simulink model "boost_converter"  (R2013a)
settings: Solver=ode23tb  StartTime=0.0  StopTime=12e-3  RelTol=1e-3
libraries: powerlib x23, powerlib_meascontrol x1
settings Model: Creator=Kevin  LastModifiedBy=kfroncza
settings DebuggingCC: SolverPrmCheckMsg=none

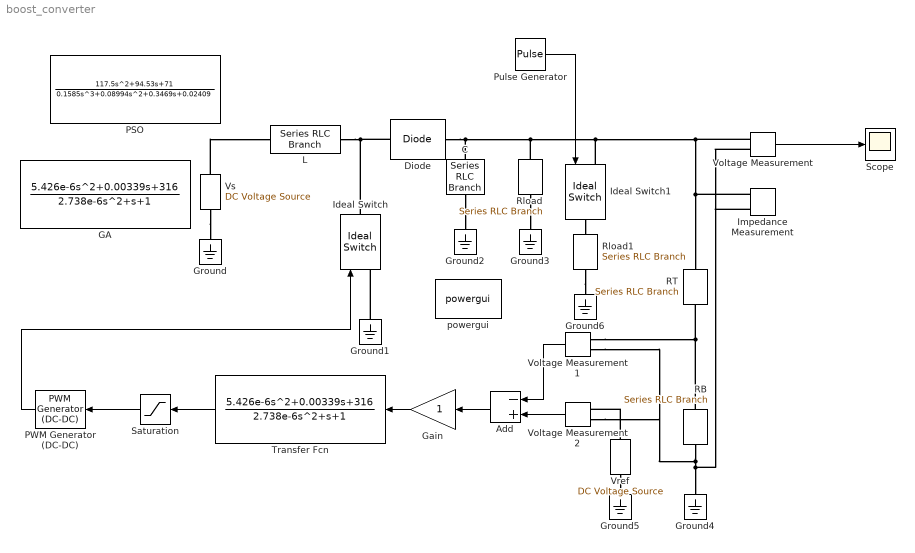
== system boost_converter ==
  Add : Sum  Inputs=-+
  C : powerlib/Elements/Series RLC Branch  LConnTagsString=__new0  RConnTagsString=__new0  BranchType=C  Resistance=1  Inductance=18e-6  SetiL0=on  InitialCurrent=0.25  Capacitance=4.7e-6  Setx0=on  InitialVoltage=5.5  Measurements=None
  Diode : powerlib/Power Electronics/Diode  Ron=0.001  Lon=0  Vf=0.1  IC=0  UseSnubber=off  Rs=500  Cs=250e-9  Measurements=off
  GA : TransferFcn  Numerator=[5.426e-6 0.00339 316]  Denominator=[2.738e-6 1 1]
  Gain : Gain
  Ground{,1..6} (7 alike) : powerlib/Elements/Ground  LConnTagsString=a
  Ideal Switch : powerlib/Power Electronics/Ideal Switch  Ron=0.001  Lon=0  IC=0  Rs=1e5  Cs=inf  Measurements=off
  Ideal Switch1 : powerlib/Power Electronics/Ideal Switch  Ron=0.001  Lon=0  IC=0  Rs=1e5  Cs=inf  Measurements=off
  Impedance Measurement : powerlib/Measurements/Impedance Measurement  LConnTagsString=+|-  Factor=1
  L : powerlib/Elements/Series RLC Branch  LConnTagsString=__new0  RConnTagsString=__new0  BranchType=L  Resistance=1  Inductance=18e-6  SetiL0=off  InitialCurrent=0  Capacitance=1e-6  Setx0=off  InitialVoltage=0  Measurements=None
  PSO : TransferFcn  Numerator=[117.5 94.53 71]  Denominator=[0.1585 0.08994 0.3469 0.02409]
  PWM Generator (DC-DC) : powerlib_meascontrol/Pulse & Signal Generators/PWM Generator (DC-DC)  Fsw=350e3  Ts=0
  Pulse Generator : DiscretePulseGenerator  PulseType=Time based  Period=8e-3
  RB : powerlib/Elements/Series RLC Branch  LConnTagsString=__new0  RConnTagsString=__new0  BranchType=R  Resistance=1.3e6  Inductance=18e-6  SetiL0=on  InitialCurrent=0.25  Capacitance=1e-6  Setx0=off  InitialVoltage=0  Measurements=None
  RT : powerlib/Elements/Series RLC Branch  LConnTagsString=__new0  RConnTagsString=__new0  BranchType=R  Resistance=4.65e6  Inductance=18e-6  SetiL0=on  InitialCurrent=0.25  Capacitance=1e-6  Setx0=off  InitialVoltage=0  Measurements=None
  Rload : powerlib/Elements/Series RLC Branch  LConnTagsString=__new0  RConnTagsString=__new0  BranchType=R  Resistance=300  Inductance=18e-6  SetiL0=on  InitialCurrent=0.25  Capacitance=1e-6  Setx0=off  InitialVoltage=0  Measurements=None
  Rload1 : powerlib/Elements/Series RLC Branch  LConnTagsString=__new0  RConnTagsString=__new0  BranchType=R  Resistance=100  Inductance=18e-6  SetiL0=on  InitialCurrent=0.25  Capacitance=1e-6  Setx0=off  InitialVoltage=0  Measurements=None
  Saturation : Saturate  UpperLimit=0.6  LowerLimit=0
  Scope : Scope
      settings: YMin=3.25  YMax=5.75  SaveName=sim_vout
  Transfer Fcn : TransferFcn  Numerator=[5.426e-6 0.00339 316]  Denominator=[2.738e-6 1 1]
  Voltage Measurement : powerlib/Measurements/Voltage Measurement  PhasorSimulation=off  OutputType=Complex  PSBequivalent=0
  Voltage Measurement1 : powerlib/Measurements/Voltage Measurement  PhasorSimulation=off  OutputType=Complex  PSBequivalent=0
  Voltage Measurement2 : powerlib/Measurements/Voltage Measurement  PhasorSimulation=off  OutputType=Complex  PSBequivalent=0
  Vref : powerlib/Electrical Sources/DC Voltage Source  Amplitude=1.2  Measurements=None
  Vs : powerlib/Electrical Sources/DC Voltage Source  Amplitude=2.75  Measurements=None
  powergui : powerlib/powergui  Priority=1  SimulationMode=Continuous  SolverType=Tustin  SampleTime=50e-6  frequency=60  SPID=off  DisableSnubberDevices=off  DisableRonSwitches=off  DisableVfSwitches=off  SwTol=0  Interpol=off  DisplayEquations=off  frequencyindice=0  Pbase=100e6  ErrMax=1e-4  Iterations=50  UnitsV=kV  UnitsW=MW  FunctionMessages=off  echomessages=off  HookPort=off  EnableUseOfTLC=off  x0status=blocks  RestoreLinks=warning  ResistiveCurrentMeasurement=off  Frange=[0:2:500]  Ylog=off  Xlog=on  ShowGrid=on  save=off  variable=ZData  ZoomFFT=on  StartTime=0.0  cycles=1  DisplayStyle=1  fundamental=60  FreqAxis=off  MaxFrequency=1000  frequencyindicesteady=1  RmsSteady=1  display=off  Ts=0  methode=off
  wires:
  Voltage Measurement2/1 -> Add/2
  Add/1 -> Gain/1
  Gain/1 -> Transfer Fcn/1
  Voltage Measurement1/1 -> Add/1
  Pulse Generator/1 -> Ideal Switch1/1
  Voltage Measurement/1 -> Scope/1
  PWM Generator (DC-DC)/1 -> Ideal Switch/1
  Saturation/1 -> PWM Generator (DC-DC)/1
  Transfer Fcn/1 -> Saturation/1
  connections:
  L/RConn1 -- Ideal Switch/RConn1 -- Diode/LConn1
  Diode/RConn1 -- Rload/LConn1 -- Ideal Switch1/LConn1 -- Voltage Measurement/LConn1 -- Impedance Measurement/LConn1 -- RT/LConn1 -- C/LConn1
  Vs/RConn1 -- L/LConn1
  RB/RConn1 -- Voltage Measurement1/LConn2 -- Voltage Measurement2/LConn2 -- Impedance Measurement/LConn2 -- Voltage Measurement/LConn2 -- Ground4/LConn1
  RB/LConn1 -- Voltage Measurement1/LConn1 -- RT/RConn1
  Rload/RConn1 -- Ground3/LConn1
  C/RConn1 -- Ground2/LConn1
  Vs/LConn1 -- Ground/LConn1
  Ground1/LConn1 -- Ideal Switch/LConn1
  Vref/LConn1 -- Ground5/LConn1
  Vref/RConn1 -- Voltage Measurement2/LConn1
  Rload1/RConn1 -- Ground6/LConn1
  Ideal Switch1/RConn1 -- Rload1/LConn1
